simulink model "Simulink_PLC_coder_example_LAB_11_simulator"  (R2023b)
settings: Solver=FixedStepDiscrete  StartTime=0.0  StopTime=10  FixedStep=0.0001  RelTol=1e-3
undefined symbols (not defined in the file): DiscIntNeverNeededParam
settings Model: Creator=Jan Størbu  LastModifiedBy=hagen
settings SolverCC: AlgebraicLoopSolver=TrustRegion
settings DataIOCC: ReturnWorkspaceOutputs=off
settings DebuggingCC: UnconnectedInputMsg=warning  UnconnectedOutputMsg=warning  UnconnectedLineMsg=warning  BusObjectLabelMismatch=error  ArithmeticOperatorsInVariantConditions=warning
settings ModelReferenceCC: EnableRefExpFcnMdlSchedulingChecks=on
settings SFSimCC: SimUseLocalCustomCode=off  CustomCodeUndefinedFunction=UseInterfaceOnly
settings RTWCC: RTWUseLocalCustomCode=off  DLArmComputeVersion=19.05
settings ConfigComp: PLC_TargetIDE=plcopen  PLC_MultiTBSigbuilderTimeRange=off  PLC_ReuseMLFcnVariable=on  PLC_FoldFBCallOutputVar=off  PLC_RemoveUnusedSSMethodCallArguments=off  PLC_UseCallOutputArgSyntax=off  PLC_EnableUnsignedAndDoubleTypes=off  PLC_EnableUDTSplitting=off  PLC_MaxFieldsInUDT=500  PLC_InlineEnumCastFunction=off  PLC_GenerateReport=off  PLC_LaunchReport=off

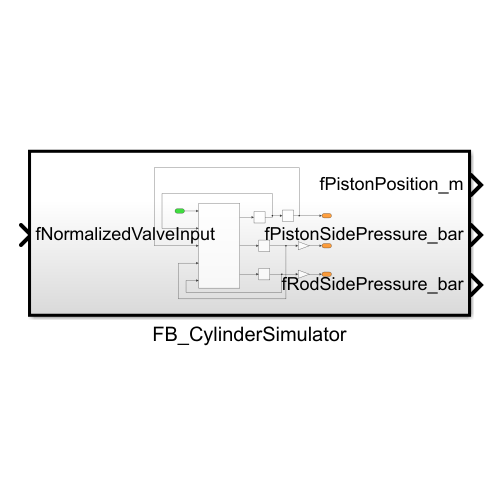
[thumbnail: Simulink's stored preview of the top-level diagram]
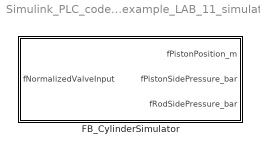
== system Simulink_PLC_coder_example_LAB_11_simulator ==
  FB_CylinderSimulator : Subsystem  TreatAsAtomicUnit=on

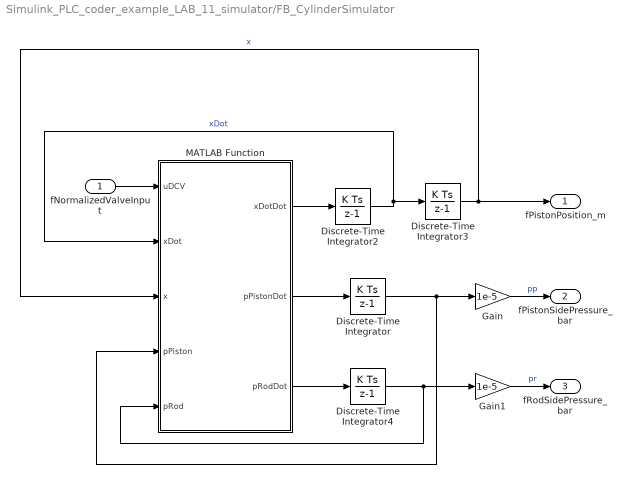
== system Simulink_PLC_coder_example_LAB_11_simulator/FB_CylinderSimulator ==
  fNormalizedValveInput : Inport
  Discrete-Time Integrator : DiscreteIntegrator  InitialCondition=68.74e5  SampleTime=-1  LimitOutput=on  UpperSaturationLimit=180e5  LowerSaturationLimit=1.1e5  ICPrevOutput=DiscIntNeverNeededParam  ICPrevScaledInput=DiscIntNeverNeededParam
  Discrete-Time Integrator2 : DiscreteIntegrator  SampleTime=-1  UpperSaturationLimit=0.12  LowerSaturationLimit=-0.12  ICPrevOutput=DiscIntNeverNeededParam  ICPrevScaledInput=DiscIntNeverNeededParam
  Discrete-Time Integrator3 : DiscreteIntegrator  SampleTime=-1  LimitOutput=on  UpperSaturationLimit=0.5  LowerSaturationLimit=0  ICPrevOutput=DiscIntNeverNeededParam  ICPrevScaledInput=DiscIntNeverNeededParam
  Discrete-Time Integrator4 : DiscreteIntegrator  InitialCondition=5.144e5  SampleTime=-1  LimitOutput=on  UpperSaturationLimit=180e5  LowerSaturationLimit=1.1e5  ICPrevOutput=DiscIntNeverNeededParam  ICPrevScaledInput=DiscIntNeverNeededParam
  Gain : Gain  Gain=1e-5
  Gain1 : Gain  Gain=1e-5
  MATLAB Function : MATLAB Function  TreatAsAtomicUnit=on
  fPistonPosition_m : Outport
  fPistonSidePressure_bar : Outport  Port=2
  fRodSidePressure_bar : Outport  Port=3
  wires:
  fNormalizedValveInput/1 -> MATLAB Function/1(uDCV)
  MATLAB Function/2(pPistonDot) -> Discrete-Time Integrator/1
  Discrete-Time Integrator3/1 -> fPistonPosition_m/1, MATLAB Function/3(x)  "x"
  Discrete-Time Integrator/1 -> Gain/1, MATLAB Function/4(pPiston)
  Discrete-Time Integrator2/1 -> Discrete-Time Integrator3/1, MATLAB Function/2(xDot)  "xDot"
  Discrete-Time Integrator4/1 -> Gain1/1, MATLAB Function/5(pRod)
  Gain/1 -> fPistonSidePressure_bar/1  "pp"
  MATLAB Function/3(pRodDot) -> Discrete-Time Integrator4/1
  MATLAB Function/1(xDotDot) -> Discrete-Time Integrator2/1
  Gain1/1 -> fRodSidePressure_bar/1  "pr"

== matlab function Simulink_PLC_coder_example_LAB_11_simulator/FB_CylinderSimulator/MATLAB Function ==
  data: uDCV input; xDot input; xDotDot output; x input; pPiston input; pRod input; pPistonDot output; pRodDot output
function [xDotDot, pPistonDot, pRodDot] = fcn(uDCV, xDot, x, pPiston, pRod)
%% Parameters
mEffective = 1.5e+04;  % [kg]
Fexternal = 2.15e+04; % [N]
kFric = 10000; % [N/(ms)]
Apiston = 0.0033; % [m^2]
Aannulus = 0.0023; % [m^2]
beta = 1.0e9; % [Pa]
pSupply = 180e5; % [Pa]
pReturn = 1.1e5; % [Pa]
MaxStroke = 0.5; % [m]
VCyl_A = 1.0e-03; 
VCyl_B = 1.25e-03; 
p_nom_DCV = 7e5;  
Q1_ref_DCV = 19/6e4;
Q2_ref_DCV = 8/6e4;
kv1_DCV = Q1_ref_DCV/sqrt(p_nom_DCV);
kv2_DCV = Q2_ref_DCV/sqrt(p_nom_DCV);
p0 = 7e5; %compensator crack pressure
%% Directional Control Valve - Lifting Cylinder 
% LS Pressure
if uDCV > 0 
     pLS = pPiston;
 elseif uDCV < 0
     pLS = pRod;
 else 
     pLS = 0;
end
 
if pLS<0
    pLS = 0;
end

% Pressure Compensator
pPC = 0;

if p0 <= (pSupply - pLS) 
      pPC = pLS+p0; 
  elseif 0 < (pSupply - pLS) < p0
        pPC = pSupply-pLS;   
  elseif (pSupply - pLS) <= 0     
      pPC = pLS;
end

 if pPC<0
     pPC = 0;
 end
% Orifice Equations
if uDCV > 0
QDCV_in =  kv1_DCV*uDCV*sign(pPC-pPiston)*sqrt(abs(pPC-pPiston)); % QpistonSide
QDCV_out = kv2_DCV*uDCV*sign(pRod-pReturn)*sqrt(abs(pRod-pReturn)); % QrodSide
elseif uDCV < 0  
QDCV_out =  kv1_DCV*uDCV*sign(pPC-pRod)*sqrt(abs(pPC-pRod)); % QrodSide
QDCV_in =  kv2_DCV*uDCV*sign(pPiston-pReturn)*sqrt(abs(pPiston-pReturn)); % QpistonSide
else
QDCV_in = 0;
QDCV_out = 0;
end
%% Pressure Gradients
VA = VCyl_A + x*Apiston;
VB =  VCyl_B + (MaxStroke - x)*Aannulus; 
VA_dot = Apiston*xDot;
VB_dot = Aannulus*xDot;
pPistonDot = beta/VA*(QDCV_in - VA_dot);
pRodDot = beta/VB*(VB_dot-QDCV_out);

% Viscouse Friction
Ffric = kFric*xDot;
%% Hydraulic Force
Fhyd = pPiston*Apiston - pRod*Aannulus;

%% Newton Second Law of Motion
xDotDot = (Fhyd - Ffric - Fexternal)/mEffective;
